simulink model "Simu_LC_Case_VI"  (R2018a)
settings: Solver=ode45  StartTime=0.0  StopTime=Map_Data.simu_time  RelTol=1e-3
values from neighbouring files (symbols this model uses):
  Map_Data = create_map(Global_Data)    [main.m]
undefined symbols (not defined in the file or in its folder): Auto
libraries: ModC_Planner x1, ModD_Controladores x1, ModG_Vehiculo x1, simulink x1
settings Model: Creator=Lisandro Cocca  LastModifiedBy=Lisandro Cocca

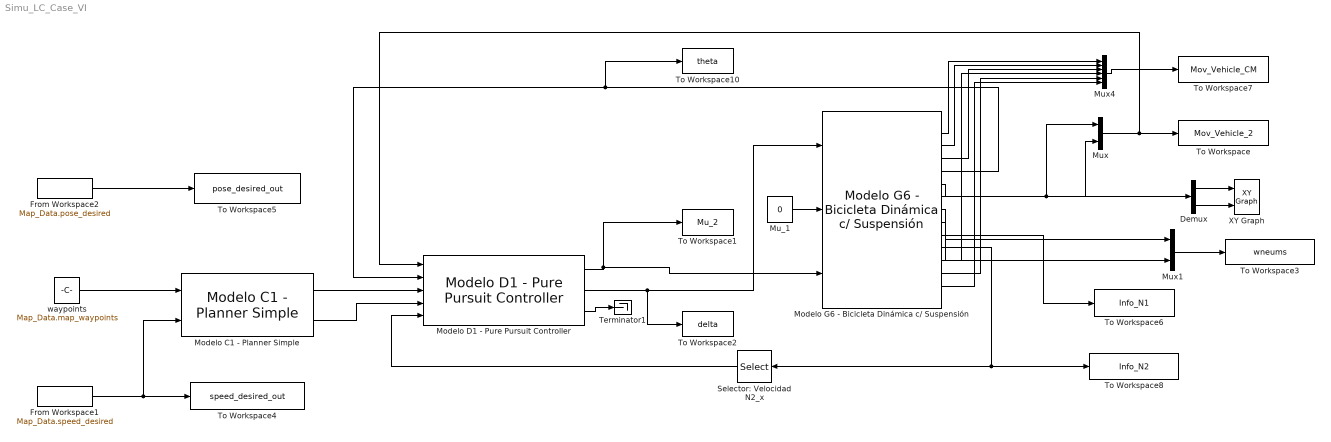
== system Simu_LC_Case_VI ==
  Demux : Demux  Outputs=2
  From Workspace1 : FromWorkspace  VariableName=Map_Data.speed_desired  SampleTime=0  Interpolate=off  OutputAfterFinalValue=Setting to zero
  From Workspace2 : FromWorkspace  VariableName=Map_Data.pose_desired  SampleTime=0  Interpolate=off  OutputAfterFinalValue=Setting to zero
  Modelo C1 - Planner Simple : ModC_Planner/Modelo C1 - Planner Simple
      settings: SourceProductName=Proyecto_Final
  "Modelo D1 - Pure Pursuit Controller " : ModD_Controladores/Modelo D1 - Pure Pursuit Controller   kla=PP_Controller.kla  L=Auto.L  la_low=PP_Controller.la_low  psi_max=Auto.psi_max
      link override Memory1: InitialCondition=2200
      settings: SourceProductName=Proyecto_Final
  Modelo G6 - Bicicleta Dinámica c/ Suspensión : ModG_Vehiculo/Modelo G6 - Bicicleta Dinámica c// Suspensión  m=Auto.m  Izz=Auto.Izz  Iyy=Auto.Iyy  L=Auto.L  a2=Auto.a2  a1=Auto.a1  g=9.81  GR=Auto.GR  Rg=Neum.Rg  Jw=Neum.Jw  k_sus=Auto.k_sus  b_sus=Auto.b_sus  h=Auto.h
      settings: SourceProductName=Proyecto_Final
  Mu_1 : Constant  Value=0  VectorParams1D=off
  Mux : Mux  Inputs=2
  Mux1 : Mux  Inputs=2
  Mux4 : Mux  Inputs=6
  Selector: Velocidad N2_x : Selector  IndexOptions=Index vector (dialog)  Indices=[1]  OutputSizes=1
  Terminator1 : Terminator
  To Workspace : ToWorkspace  VariableName=Mov_Vehicle_2  SampleTime=-1
  To Workspace1 : ToWorkspace  VariableName=Mu_2  SampleTime=-1
  To Workspace10 : ToWorkspace  VariableName=theta  SampleTime=-1
  To Workspace2 : ToWorkspace  VariableName=delta  SampleTime=-1
  To Workspace3 : ToWorkspace  VariableName=wneums  SampleTime=-1
  To Workspace4 : ToWorkspace  VariableName=speed_desired_out  SampleTime=-1
  To Workspace5 : ToWorkspace  VariableName=pose_desired_out  SampleTime=-1
  To Workspace6 : ToWorkspace  VariableName=Info_N1  SampleTime=-1
  To Workspace7 : ToWorkspace  VariableName=Mov_Vehicle_CM  SampleTime=-1
  To Workspace8 : ToWorkspace  VariableName=Info_N2  SampleTime=-1
  XY Graph : simulink/Sinks/XY Graph  xmin=-5  xmax=10  ymin=-5  ymax=10  st=-1
  "waypoints " : Constant  Value=Map_Data.map_waypoints  VectorParams1D=off
  wires:
  "Modelo D1 - Pure Pursuit Controller "/2 -> Modelo G6 - Bicicleta Dinámica c/ Suspensión/1, To Workspace2/1
  "Modelo D1 - Pure Pursuit Controller "/1 -> Modelo G6 - Bicicleta Dinámica c/ Suspensión/3, To Workspace1/1
  "waypoints "/1 -> Modelo C1 - Planner Simple/1
  From Workspace1/1 -> To Workspace4/1, Modelo C1 - Planner Simple/2
  Modelo C1 - Planner Simple/2 -> "Modelo D1 - Pure Pursuit Controller "/4
  Modelo C1 - Planner Simple/1 -> "Modelo D1 - Pure Pursuit Controller "/3
  Demux/1 -> XY Graph/1
  Demux/2 -> XY Graph/2
  Mux/1 -> "Modelo D1 - Pure Pursuit Controller "/1, To Workspace/1
  Selector: Velocidad N2_x/1 -> "Modelo D1 - Pure Pursuit Controller "/5
  Mu_1/1 -> Modelo G6 - Bicicleta Dinámica c/ Suspensión/2
  Modelo G6 - Bicicleta Dinámica c/ Suspensión/5 -> Mux/1, Demux/1
  Modelo G6 - Bicicleta Dinámica c/ Suspensión/4 -> To Workspace10/1, "Modelo D1 - Pure Pursuit Controller "/2
  "Modelo D1 - Pure Pursuit Controller "/3 -> Terminator1/1
  Mux4/1 -> To Workspace7/1
  From Workspace2/1 -> To Workspace5/1
  Modelo G6 - Bicicleta Dinámica c/ Suspensión/6 -> Mux/2
  Modelo G6 - Bicicleta Dinámica c/ Suspensión/1 -> Mux4/1
  Modelo G6 - Bicicleta Dinámica c/ Suspensión/2 -> Mux4/2
  Modelo G6 - Bicicleta Dinámica c/ Suspensión/3 -> Mux4/3
  Modelo G6 - Bicicleta Dinámica c/ Suspensión/7 -> Mux1/1
  Modelo G6 - Bicicleta Dinámica c/ Suspensión/8 -> Mux1/2
  Mux1/1 -> To Workspace3/1
  Modelo G6 - Bicicleta Dinámica c/ Suspensión/10 -> To Workspace8/1, Selector: Velocidad N2_x/1
  Modelo G6 - Bicicleta Dinámica c/ Suspensión/9 -> To Workspace6/1
  Modelo G6 - Bicicleta Dinámica c/ Suspensión/11 -> Mux4/4
  Modelo G6 - Bicicleta Dinámica c/ Suspensión/12 -> Mux4/5
  Modelo G6 - Bicicleta Dinámica c/ Suspensión/13 -> Mux4/6
